simulink model "ev_phase1"  (R2025a)
settings: Solver=VariableStepAuto  StartTime=0.0  StopTime=2  RelTol=1e-3
settings Model: Creator=piyus  LastModifiedBy=piyus

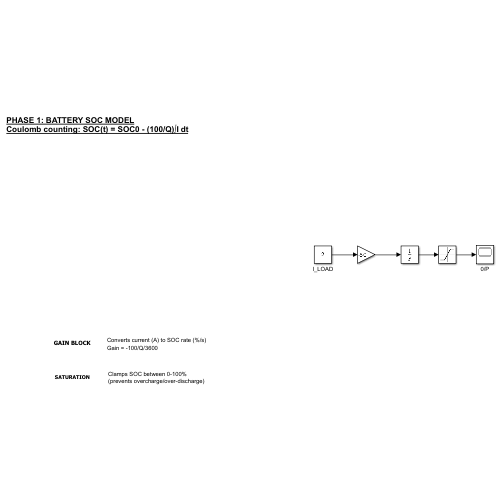
[thumbnail: Simulink's stored preview of the top-level diagram]
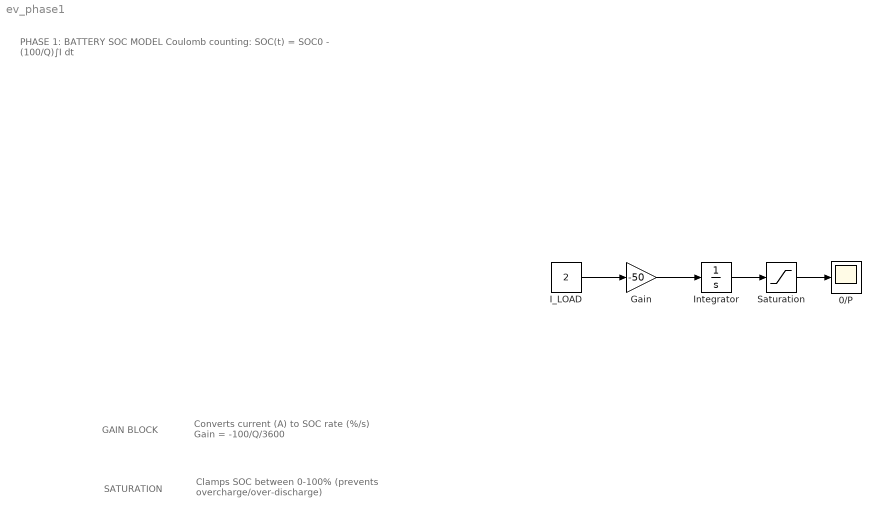
== system ev_phase1 ==
  note: SATURATION
  note: GAIN BLOCK
  note: Clamps SOC between 0-100%
      | (prevents overcharge/over-discharge)
  note: Converts current (A) to SOC rate (%/s)
      | Gain = -100/Q/3600
  note: PHASE 1: BATTERY SOC MODEL
      | Coulomb counting: SOC(t) = SOC0 - (100/Q)∫I dt
  0/P : Scope
      settings: ActiveDisplayYMinimum=-124.65492788290996  ActiveDisplayYMaximum=150.97007211708981
  Gain : Gain  Gain=-50
  I_LOAD : Constant  Value=2
  Integrator : Integrator  InitialCondition=100
  Saturation : Saturate  UpperLimit=100  LowerLimit=0
  wires:
  I_LOAD/1 -> Gain/1
  Gain/1 -> Integrator/1
  Integrator/1 -> Saturation/1
  Saturation/1 -> 0/P/1
